simulink model "NL_Simulation"  (R2018b)
settings: Solver=VariableStepAuto  StartTime=0.0  StopTime=12.4  FixedStep=0.01
model workspace: external: MAT-File /home/abhineet/Research/Nonlinear_Model/Simulation_6dof/NL_Sim/setup_NL.mat (data not in the file)
values from neighbouring files (symbols this model uses):
  StateVals = SetInitial(Vinf,AeroType)    [setup_NL.m]
undefined symbols (not defined in the file or in its folder): AC, Mass
libraries: Tools_6dofSimulation x24, aerolibasang x3, dspmathops x3, shared6dofsys x2, shared6dof x2, aerolibatmos2 x1, sharedtransform x1, sharedutil x1
(part 2 of 2)

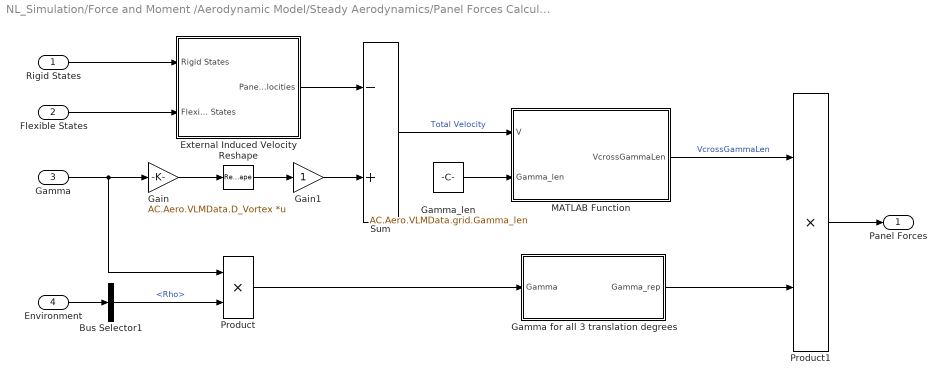
== system NL_Simulation/Force and Moment /Aerodynamic Model/Steady Aerodynamics/Panel Forces Calculation ==
  Rigid States : Inport
  Flexible States : Inport  Port=2
  Gamma : Inport  Port=3
  Environment : Inport  Port=4
  Bus Selector1 : BusSelector  OutputSignals=Rho
  External Induced Velocity : Subsystem
  Gain : Gain  Gain=AC.Aero.VLMData.D_Vortex  Multiplication=Matrix(K*u)
  Gain1 : Gain
  Gamma for all 3 translation degrees : MATLAB Function  TreatAsAtomicUnit=on
  Gamma_len : Constant  Value=AC.Aero.VLMData.grid.Gamma_len
  MATLAB Function : MATLAB Function  TreatAsAtomicUnit=on
  Product : Product
  Product1 : Product
  Reshape : Reshape  OutputDimensionality=Customize  OutputDimensions=[3,AC.Aero.NumPanels]
  Sum : Sum  Inputs=-+
  Panel Forces : Outport
  wires:
  Rigid States/1 -> External Induced Velocity/1(Rigid States)
  Flexible States/1 -> External Induced Velocity/2(Flexible States)
  External Induced Velocity/1(Panel Velocities) -> Sum/1
  Environment/1 -> Bus Selector1/1
  Gain/1 -> Reshape/1
  Reshape/1 -> Gain1/1
  Gamma/1 -> Gain/1, Product/1
  Sum/1 -> MATLAB Function/1(V)  "Total Velocity"
  Gamma_len/1 -> MATLAB Function/2(Gamma_len)
  Bus Selector1/1 -> Product/2  "<Rho>"
  Product/1 -> Gamma for all 3 translation degrees/1(Gamma)
  Gamma for all 3 translation degrees/1(Gamma_rep) -> Product1/2
  Product1/1 -> Panel Forces/1
  MATLAB Function/1(VcrossGammaLen) -> Product1/1  "VcrossGammaLen"
  Gain1/1 -> Sum/2

== system NL_Simulation/Force and Moment /Aerodynamic Model/Steady Aerodynamics/Total Wash ==
  note: The rigid body states are first transformed into Aerodynamic Axes and used to calculate total wash. Note that the calculated total wash is same as the internal wash generated by the vortices.
  Rigid States : Inport
  Flexible States : Inport  Port=2
  Bus Selector : BusSelector  OutputSignals=Vb,Omegab
  Flexible defections : Subsystem
  Gain : Gain  Gain=[-1,1,-1]
  Gain1 : Gain  Gain=[-1,1,-1]
  Repmat function : MATLAB Function  TreatAsAtomicUnit=on  mask{NumPanels=AC.Aero.NumPanels}
      mask prompts: NumPanels "Number of Panels"
      mask init:
      | % NumPanels = 888;
  Sum : Sum  Inputs=+++
  Vel_Omega : Subsystem
  Total  Wash : Outport
  wires:
  Rigid States/1 -> Bus Selector/1
  Bus Selector/1 -> Gain/1  "<Vb>"
  Bus Selector/2 -> Gain1/1  "<Omegab>"
  Vel_Omega/1(Omegacrossr) -> Sum/2
  Gain/1 -> Repmat function/1(V)
  Gain1/1 -> Vel_Omega/1(Omegab)
  Flexible States/1 -> Flexible defections/1(Flexible States)
  Flexible defections/1(Del_r_flex) -> Vel_Omega/2(Del_r_flex)
  Flexible defections/2(Del_v_flex) -> Sum/3
  Sum/1 -> Total  Wash/1
  Repmat function/1(Vrepmat) -> Sum/1

== system NL_Simulation/Force and Moment /Aerodynamic Model/Steady Aerodynamics/Vortex Strength ==
  Flexible States : Inport
  Normal wash : Inport  Port=2
  AIC Calculation : Subsystem
  Product : Product  Multiplication=Matrix(*)
  Gamma : Outport
  wires:
  Product/1 -> Gamma/1
  Flexible States/1 -> AIC Calculation/1(Flexible States)
  AIC Calculation/1(AIC) -> Product/1
  Normal wash/1 -> Product/2  "Normal wash"

== system NL_Simulation/Force and Moment /Aerodynamic Model/Unsteady Aerodynamics/Normal Forces ==
  Normal Wash Derivatives : Inport
  Rigid States : Inport  Port=2
  Gain : Gain  Gain=AC.Aero.DLMData.A1  Multiplication=Matrix(K*u)
  Gain1 : Gain  Gain=AC.Aero.DLMData.Clag  Multiplication=Matrix(K*u)
  MACby2V : Subsystem
  Product : Product
  Subsystem1 : Subsystem
  Sum : Sum
  Normal Forces : Outport
  wires:
  Normal Wash Derivatives/1 -> Product/1
  Sum/1 -> Normal Forces/1
  Rigid States/1 -> MACby2V/1(Rigid States)
  MACby2V/1(MACby2V) -> Product/2, Subsystem1/2(b_over_V)
  Product/1 -> Subsystem1/1(Normal Wash Derivative), Gain/1
  Gain/1 -> Sum/1
  Subsystem1/1(Lag States) -> Gain1/1
  Gain1/1 -> Sum/2

== system NL_Simulation/Force and Moment /Aerodynamic Model/Unsteady Aerodynamics/Normal Wash Derivative ==
  Total Wash Derivative : Inport
  Constant : Constant  Value=AC.Aero.Nhat0
  Product : Product
  Sum : Sum  Inputs=+  CollapseMode=Specified dimension
  Transpose : Math  Operator=transpose  SaturateOnIntegerOverflow=on
  Normal Wash Derivative : Outport
  wires:
  Sum/1 -> Transpose/1
  Constant/1 -> Product/1
  Total Wash Derivative/1 -> Product/2
  Product/1 -> Sum/1
  Transpose/1 -> Normal Wash Derivative/1

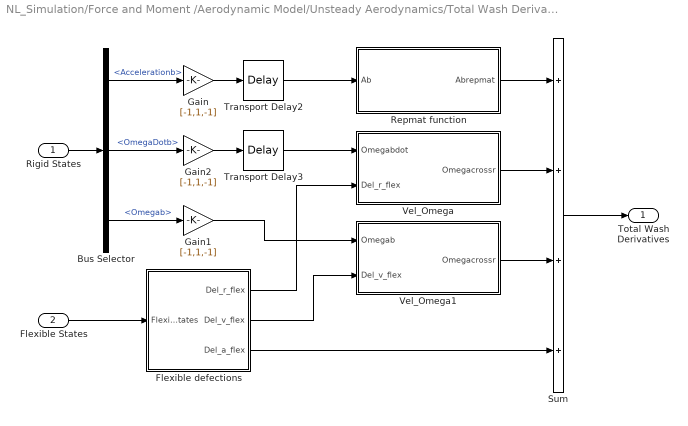
== system NL_Simulation/Force and Moment /Aerodynamic Model/Unsteady Aerodynamics/Total Wash Derivative ==
  Rigid States : Inport
  Flexible States : Inport  Port=2
  Bus Selector : BusSelector  OutputSignals=Accelerationb,OmegaDotb,Omegab
  Flexible defections : Subsystem
  Gain : Gain  Gain=[-1,1,-1]
  Gain1 : Gain  Gain=[-1,1,-1]
  Gain2 : Gain  Gain=[-1,1,-1]
  Repmat function : MATLAB Function  TreatAsAtomicUnit=on  mask{NumPanels=AC.Aero.NumPanels}
      mask prompts: NumPanels "Number of Panels"
      mask init:
      | % NumPanels = 888;
  Sum : Sum  Inputs=++++
  Transport Delay2 : TransportDelay  DelayTime=0.001  PadeOrder=2
  Transport Delay3 : TransportDelay  DelayTime=0.001  PadeOrder=2
  Vel_Omega : Subsystem
  Vel_Omega1 : Subsystem
  Total Wash Derivatives : Outport
  wires:
  Rigid States/1 -> Bus Selector/1
  Bus Selector/1 -> Gain/1  "<Accelerationb>"
  Vel_Omega/1(Omegacrossr) -> Sum/2
  Gain2/1 -> Transport Delay3/1
  Flexible States/1 -> Flexible defections/1(Flexible States)
  Sum/1 -> Total Wash Derivatives/1
  Repmat function/1(Abrepmat) -> Sum/1
  Bus Selector/2 -> Gain2/1  "<OmegaDotb>"
  Flexible defections/2(Del_v_flex) -> Vel_Omega1/2(Del_v_flex)
  Vel_Omega1/1(Omegacrossr) -> Sum/3
  Flexible defections/1(Del_r_flex) -> Vel_Omega/2(Del_r_flex)
  Gain/1 -> Transport Delay2/1
  Flexible defections/3(Del_a_flex) -> Sum/4
  Bus Selector/3 -> Gain1/1  "<Omegab>"
  Gain1/1 -> Vel_Omega1/1(Omegab)
  Transport Delay2/1 -> Repmat function/1(Ab)
  Transport Delay3/1 -> Vel_Omega/1(Omegabdot)

== system NL_Simulation/Sensors1/Sensors/Accelerometer Rigid/Vel_Omega ==
  Omegabdot : Inport
  Cross Product Matrix : Tools_6dofSimulation/Cross Product Matrix  SystemSampleTime=-1
  Demux : Demux  Outputs=3
  Product : Product  Multiplication=Matrix(*)
  rcg_sensor : Constant  Value=AC.SensorData.SensorAeroGrid
  Omegabcrossr : Outport
  wires:
  Omegabdot/1 -> Demux/1
  Product/1 -> Omegabcrossr/1
  Demux/2 -> Cross Product Matrix/2  "qdot"
  Demux/3 -> Cross Product Matrix/3  "rdot"
  Cross Product Matrix/1 -> Product/1
  rcg_sensor/1 -> Product/2
  Demux/1 -> Cross Product Matrix/1  "pdot"

== system NL_Simulation/Sensors1/Sensors/Accelerometer Rigid/Vel_Omega2 ==
  Omegabdot : Inport
  Cross Product Matrix : Tools_6dofSimulation/Cross Product Matrix  SystemSampleTime=-1
  Demux : Demux  Outputs=3
  Product : Product  Multiplication=Matrix(*)
  Product1 : Product  Multiplication=Matrix(*)
  rcg_sensor : Constant  Value=AC.SensorData.SensorAeroGrid
  Omegabcrossr : Outport
  wires:
  Omegabdot/1 -> Demux/1
  Demux/2 -> Cross Product Matrix/2  "qdot"
  Demux/3 -> Cross Product Matrix/3  "rdot"
  Cross Product Matrix/1 -> Product1/1, Product/1
  rcg_sensor/1 -> Product/2
  Demux/1 -> Cross Product Matrix/1  "pdot"
  Product/1 -> Product1/2
  Product1/1 -> Omegabcrossr/1

== system NL_Simulation/Sensors1/Sensors/Accelerometers/Flexible defections ==
  Flexible States : Inport
  Bus Selector1 : BusSelector  OutputSignals=EtaFlex,EtaFlexdot,EtaFlexdotdot
  Phif_Translation : Constant  Value=AC.ModalStruc.Phif_aero_sensor_Trans  VectorParams1D=off
  Product1 : Product  Multiplication=Matrix(*)
  Product2 : Product  Multiplication=Matrix(*)
  Product3 : Product  Multiplication=Matrix(*)
  Reshape1 : Reshape  OutputDimensionality=Customize  OutputDimensions=[3,AC.SensorData.NumSensors]
  Reshape2 : Reshape  OutputDimensionality=Customize  OutputDimensions=[3,AC.SensorData.NumSensors]
  Reshape3 : Reshape  OutputDimensionality=Customize  OutputDimensions=[3,AC.SensorData.NumSensors]
  Del_r_flex : Outport
  Del_v_flex : Outport  Port=2
  Del_a_flex : Outport  Port=3
  wires:
  Product1/1 -> Reshape1/1
  Bus Selector1/2 -> Product2/2  "<EtaFlexdot>"
  Reshape1/1 -> Del_r_flex/1
  Flexible States/1 -> Bus Selector1/1
  Product2/1 -> Reshape2/1
  Phif_Translation/1 -> Product3/1, Product2/1, Product1/1
  Bus Selector1/1 -> Product1/2  "<EtaFlex>"
  Reshape2/1 -> Del_v_flex/1
  Bus Selector1/3 -> Product3/2  "<EtaFlexdotdot>"
  Product3/1 -> Reshape3/1
  Reshape3/1 -> Del_a_flex/1

== system NL_Simulation/Sensors1/Sensors/Accelerometers/Subsystem ==
  In1 : Inport
  Bus Selector1 : BusSelector  OutputSignals=EtaFlex
  Gain : Gain  Gain=AC.ModalStruc.Phif_aero_sensor_Rot  Multiplication=Matrix(K*u)
  Normalization : dspmathops/Normalization  NormType=2-norm  Bias=1e-10  NormOver=Each column  Dimension=1  roundingMode=Floor  overflowMode=off  accumDataTypeStr=Inherit: Same as product output  accumLastDataTypeStr=Inherit: Same as product output  outputDataTypeStr=Inherit: Same as product output  outputMin=[]  outputMax=[]  outputLastDataTypeStr=Inherit: Same as product output
      settings: SourceProductName=DSP System Toolbox
  Reshape : Reshape  OutputDimensionality=Customize  OutputDimensions=[3,AC.SensorData.NumSensors]
  SensorOrient : Constant  Value=AC.SensorData.SensorOrientation
  Sum1 : Sum
  Out1 : Outport
  wires:
  SensorOrient/1 -> Sum1/2
  Normalization/1 -> Out1/1
  Reshape/1 -> Sum1/1
  In1/1 -> Bus Selector1/1
  Sum1/1 -> Normalization/1
  Gain/1 -> Reshape/1
  Bus Selector1/1 -> Gain/1  "<EtaFlex>"

== system NL_Simulation/Sensors1/Sensors/Accelerometers/Vel_Omega ==
  Omegabdot : Inport
  Del_r_flex : Inport  Port=2
  Cross Product Matrix : Tools_6dofSimulation/Cross Product Matrix  SystemSampleTime=-1
  Demux : Demux  Outputs=3
  Product : Product  Multiplication=Matrix(*)
  Sum : Sum
  rcg_sensor : Constant  Value=AC.SensorData.SensorAeroGrid
  Omegabcrossr : Outport
  wires:
  Omegabdot/1 -> Demux/1
  Product/1 -> Omegabcrossr/1
  Demux/2 -> Cross Product Matrix/2  "qdot"
  Demux/3 -> Cross Product Matrix/3  "rdot"
  Cross Product Matrix/1 -> Product/1
  Sum/1 -> Product/2
  Del_r_flex/1 -> Sum/1
  rcg_sensor/1 -> Sum/2
  Demux/1 -> Cross Product Matrix/1  "pdot"

== system NL_Simulation/Sensors1/Sensors/Accelerometers/Vel_Omega1 ==
  Omegab : Inport
  Del_v_flex : Inport  Port=2
  Cross Product Matrix : Tools_6dofSimulation/Cross Product Matrix  SystemSampleTime=-1
  Demux : Demux  Outputs=3
  Gain : Gain  Gain=2
  Product : Product  Multiplication=Matrix(*)
  TwoOmegabcrossrdot : Outport
  wires:
  Omegab/1 -> Demux/1
  Product/1 -> Gain/1
  Demux/2 -> Cross Product Matrix/2  "qdot"
  Demux/3 -> Cross Product Matrix/3  "rdot"
  Cross Product Matrix/1 -> Product/1
  Del_v_flex/1 -> Product/2
  Demux/1 -> Cross Product Matrix/1  "pdot"
  Gain/1 -> TwoOmegabcrossrdot/1

== system NL_Simulation/Sensors1/Sensors/Accelerometers/Vel_Omega2 ==
  Omegabdot : Inport
  Del_r_flex : Inport  Port=2
  Cross Product Matrix : Tools_6dofSimulation/Cross Product Matrix  SystemSampleTime=-1
  Demux : Demux  Outputs=3
  Product : Product  Multiplication=Matrix(*)
  Product1 : Product  Multiplication=Matrix(*)
  Sum : Sum
  rcg_sensor : Constant  Value=AC.SensorData.SensorAeroGrid
  Omegabcrossr : Outport
  wires:
  Omegabdot/1 -> Demux/1
  Demux/2 -> Cross Product Matrix/2  "qdot"
  Demux/3 -> Cross Product Matrix/3  "rdot"
  Cross Product Matrix/1 -> Product1/1, Product/1
  Sum/1 -> Product/2
  Del_r_flex/1 -> Sum/1
  rcg_sensor/1 -> Sum/2
  Demux/1 -> Cross Product Matrix/1  "pdot"
  Product/1 -> Product1/2
  Product1/1 -> Omegabcrossr/1

== system NL_Simulation/Flight Mechanics/Added Mass/Subsystem3/Normal Forces/MACby2V ==
  Rigid States : Inport
  Bus Selector : BusSelector  OutputSignals=Vb
  Constant : Constant  Value=AC.Aero.MAC
  Gain : Gain  Gain=.5
  Product : Product  Inputs=*/
  Vs Calculation : Subsystem
  MACby2V : Outport
  wires:
  Vs Calculation/1(Vs) -> Product/2
  Rigid States/1 -> Bus Selector/1
  Product/1 -> MACby2V/1
  Bus Selector/1 -> Vs Calculation/1(<Vb>)  "<Vb>"
  Constant/1 -> Gain/1
  Gain/1 -> Product/1

== system NL_Simulation/Flight Mechanics/Added Mass/Subsystem3/Normal Forces/Subsystem1 ==
  Normal Wash Derivative : Inport
  b_over_V : Inport  Port=2
  A_lag : Gain  Gain=AC.Aero.DLMData.Alag  Multiplication=Matrix(K*u)
  B_lag : Gain  Gain=AC.Aero.DLMData.Blag  Multiplication=Matrix(K*u)
  Lag : Integrator  InitialCondition=zeros(1776,1)
  Product : Product  Inputs=/*
  Sum : Sum  Inputs=|++
  Lag States : Outport
  wires:
  Normal Wash Derivative/1 -> B_lag/1
  B_lag/1 -> Sum/1
  Sum/1 -> Lag/1
  Lag/1 -> Product/2
  b_over_V/1 -> Product/1
  Product/1 -> A_lag/1, Lag States/1
  A_lag/1 -> Sum/2

== system NL_Simulation/Flight Mechanics/Added Mass/Subsystem3/Total Wash Derivative/Flexible defections ==
  Flexible States : Inport
  Bus Selector1 : BusSelector  OutputSignals=EtaFlex,EtaFlexdot,EtaFlexdotdot
  Phif_Translation : Constant  Value=AC.ModalStruc.Phif_aero_trans
  Product1 : Product  Multiplication=Matrix(*)
  Product2 : Product  Multiplication=Matrix(*)
  Product3 : Product  Multiplication=Matrix(*)
  Reshape1 : Reshape  OutputDimensionality=Customize  OutputDimensions=[3,AC.Aero.NumPanels]
  Reshape2 : Reshape  OutputDimensionality=Customize  OutputDimensions=[3,AC.Aero.NumPanels]
  Reshape3 : Reshape  OutputDimensionality=Customize  OutputDimensions=[3,AC.Aero.NumPanels]
  Transport Delay3 : TransportDelay  DelayTime=0.001  PadeOrder=2
  Del_r_flex : Outport
  Del_v_flex : Outport  Port=2
  Del_a_flex : Outport  Port=3
  wires:
  Product1/1 -> Reshape1/1
  Bus Selector1/2 -> Product2/2  "<EtaFlexdot>"
  Reshape1/1 -> Del_r_flex/1
  Flexible States/1 -> Bus Selector1/1
  Product2/1 -> Reshape2/1
  Bus Selector1/1 -> Product1/2  "<EtaFlex>"
  Reshape2/1 -> Del_v_flex/1
  Phif_Translation/1 -> Product3/1, Product2/1, Product1/1
  Bus Selector1/3 -> Transport Delay3/1  "<EtaFlexdotdot>"
  Product3/1 -> Reshape3/1
  Reshape3/1 -> Del_a_flex/1
  Transport Delay3/1 -> Product3/2

== system NL_Simulation/Flight Mechanics/Added Mass/Subsystem3/Total Wash Derivative/Vel_Omega ==
  Omegabdot : Inport
  Del_r_flex : Inport  Port=2
  Cross Product Matrix : Tools_6dofSimulation/Cross Product Matrix  SystemSampleTime=-1
  Demux : Demux  Outputs=3
  Product : Product  Multiplication=Matrix(*)
  Sum : Sum
  rcg_colloc : Constant  Value=AC.Aero.VLMData.grid.r_cgcolloc
  Omegacrossr : Outport
  wires:
  Omegabdot/1 -> Demux/1
  Product/1 -> Omegacrossr/1
  Demux/2 -> Cross Product Matrix/2  "q"
  Demux/3 -> Cross Product Matrix/3  "r"
  Cross Product Matrix/1 -> Product/1
  Sum/1 -> Product/2
  Del_r_flex/1 -> Sum/1
  rcg_colloc/1 -> Sum/2
  Demux/1 -> Cross Product Matrix/1  "p"

== system NL_Simulation/Flight Mechanics/Added Mass/Subsystem3/Total Wash Derivative/Vel_Omega1 ==
  Omegab : Inport
  Del_v_flex : Inport  Port=2
  Cross Product Matrix : Tools_6dofSimulation/Cross Product Matrix  SystemSampleTime=-1
  Demux : Demux  Outputs=3
  Product : Product  Multiplication=Matrix(*)
  Omegacrossr : Outport
  wires:
  Omegab/1 -> Demux/1
  Product/1 -> Omegacrossr/1
  Demux/2 -> Cross Product Matrix/2  "q"
  Demux/3 -> Cross Product Matrix/3  "r"
  Cross Product Matrix/1 -> Product/1
  Del_v_flex/1 -> Product/2
  Demux/1 -> Cross Product Matrix/1  "p"

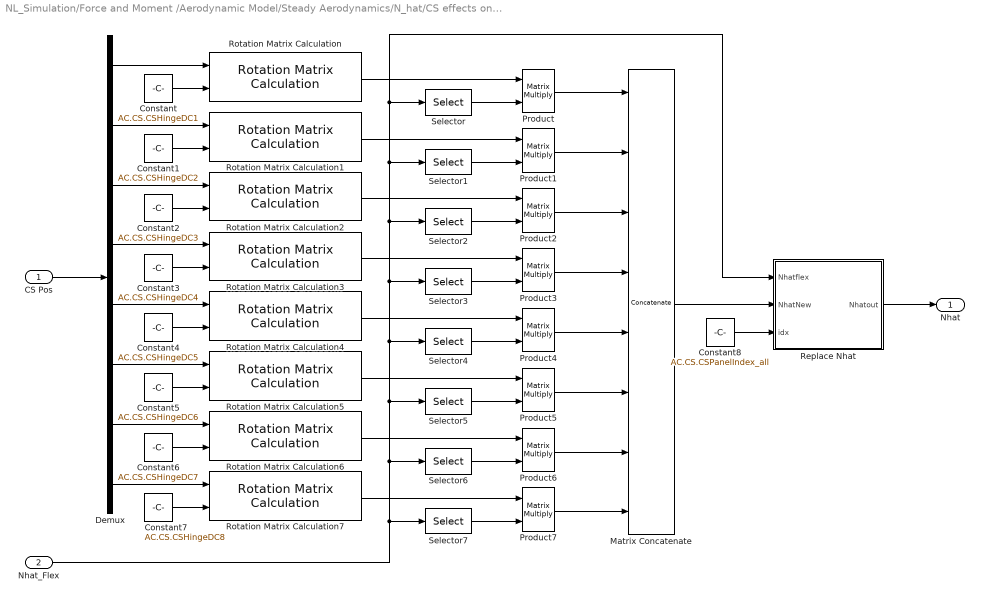
== system NL_Simulation/Force and Moment /Aerodynamic Model/Steady Aerodynamics/N_hat/CS effects on normal vectors ==
  CS Pos : Inport
  Nhat_Flex : Inport  Port=2
  Constant : Constant  Value=AC.CS.CSHingeDC1
  Constant1 : Constant  Value=AC.CS.CSHingeDC2
  Constant2 : Constant  Value=AC.CS.CSHingeDC3
  Constant3 : Constant  Value=AC.CS.CSHingeDC4
  Constant4 : Constant  Value=AC.CS.CSHingeDC5
  Constant5 : Constant  Value=AC.CS.CSHingeDC6
  Constant6 : Constant  Value=AC.CS.CSHingeDC7
  Constant7 : Constant  Value=AC.CS.CSHingeDC8
  Constant8 : Constant  Value=AC.CS.CSPanelIndex_all
  Demux : Demux  Outputs=8
  Matrix Concatenate : Concatenate  NumInputs=8  Mode=Multidimensional array  ConcatenateDimension=2
  Product{,1..7} (8 alike) : Product  Multiplication=Matrix(*)
  Replace Nhat : MATLAB Function  TreatAsAtomicUnit=on
  Rotation Matrix Calculation{,1..7} (8 alike) : Tools_6dofSimulation/Rotation Matrix Calculation  SystemSampleTime=-1
  Selector : Selector  NumberOfDimensions=2  InputPortWidth=3  IndexOptions=Select all,Index vector (dialog)  Indices=[1 3],AC.CS.CSPanelIndex1  OutputSizes=1,1
  Selector1 : Selector  NumberOfDimensions=2  InputPortWidth=3  IndexOptions=Select all,Index vector (dialog)  Indices=[1 3],AC.CS.CSPanelIndex2  OutputSizes=1,1
  Selector2 : Selector  NumberOfDimensions=2  InputPortWidth=3  IndexOptions=Select all,Index vector (dialog)  Indices=[1 3],AC.CS.CSPanelIndex3  OutputSizes=1,1
  Selector3 : Selector  NumberOfDimensions=2  InputPortWidth=3  IndexOptions=Select all,Index vector (dialog)  Indices=[1 3],AC.CS.CSPanelIndex4  OutputSizes=1,1
  Selector4 : Selector  NumberOfDimensions=2  InputPortWidth=3  IndexOptions=Select all,Index vector (dialog)  Indices=[1 3],AC.CS.CSPanelIndex5  OutputSizes=1,1
  Selector5 : Selector  NumberOfDimensions=2  InputPortWidth=3  IndexOptions=Select all,Index vector (dialog)  Indices=[1 3],AC.CS.CSPanelIndex6  OutputSizes=1,1
  Selector6 : Selector  NumberOfDimensions=2  InputPortWidth=3  IndexOptions=Select all,Index vector (dialog)  Indices=[1 3],AC.CS.CSPanelIndex7  OutputSizes=1,1
  Selector7 : Selector  NumberOfDimensions=2  InputPortWidth=3  IndexOptions=Select all,Index vector (dialog)  Indices=[1 3],AC.CS.CSPanelIndex8  OutputSizes=1,1
  Nhat : Outport
  wires:
  CS Pos/1 -> Demux/1
  Demux/1 -> Rotation Matrix Calculation/1
  Demux/2 -> Rotation Matrix Calculation1/1
  Demux/3 -> Rotation Matrix Calculation2/1
  Demux/4 -> Rotation Matrix Calculation3/1
  Demux/5 -> Rotation Matrix Calculation4/1
  Demux/6 -> Rotation Matrix Calculation5/1
  Demux/7 -> Rotation Matrix Calculation6/1
  Demux/8 -> Rotation Matrix Calculation7/1
  Constant/1 -> Rotation Matrix Calculation/2
  Constant1/1 -> Rotation Matrix Calculation1/2
  Constant2/1 -> Rotation Matrix Calculation2/2
  Constant3/1 -> Rotation Matrix Calculation3/2
  Constant4/1 -> Rotation Matrix Calculation4/2
  Constant5/1 -> Rotation Matrix Calculation5/2
  Constant6/1 -> Rotation Matrix Calculation6/2
  Constant7/1 -> Rotation Matrix Calculation7/2
  Rotation Matrix Calculation/1 -> Product/1
  Rotation Matrix Calculation1/1 -> Product1/1
  Rotation Matrix Calculation2/1 -> Product2/1
  Rotation Matrix Calculation3/1 -> Product3/1
  Rotation Matrix Calculation4/1 -> Product4/1
  Rotation Matrix Calculation6/1 -> Product6/1
  Rotation Matrix Calculation7/1 -> Product7/1
  Nhat_Flex/1 -> Replace Nhat/1(Nhatflex), Selector/1, Selector1/1, Selector2/1, Selector3/1, Selector4/1, Selector5/1, Selector6/1, Selector7/1
  Selector/1 -> Product/2
  Selector1/1 -> Product1/2
  Selector2/1 -> Product2/2
  Selector3/1 -> Product3/2
  Selector4/1 -> Product4/2
  Rotation Matrix Calculation5/1 -> Product5/1
  Selector5/1 -> Product5/2
  Selector6/1 -> Product6/2
  Selector7/1 -> Product7/2
  Constant8/1 -> Replace Nhat/3(idx)
  Product1/1 -> Matrix Concatenate/2
  Product2/1 -> Matrix Concatenate/3
  Product3/1 -> Matrix Concatenate/4
  Product4/1 -> Matrix Concatenate/5
  Product5/1 -> Matrix Concatenate/6
  Product6/1 -> Matrix Concatenate/7
  Product7/1 -> Matrix Concatenate/8
  Replace Nhat/1(Nhatout) -> Nhat/1
  Product/1 -> Matrix Concatenate/1
  Matrix Concatenate/1 -> Replace Nhat/2(NhatNew)

== system NL_Simulation/Force and Moment /Aerodynamic Model/Steady Aerodynamics/Panel Forces Calculation/External Induced Velocity ==
  Rigid States : Inport
  Flexible States : Inport  Port=2
  Bus Selector : BusSelector  OutputSignals=Vb,Omegab
  Flexible defections : Subsystem
  Gain : Gain  Gain=[-1,1,-1]
  Gain1 : Gain  Gain=[-1,1,-1]
  Repmat function : MATLAB Function  TreatAsAtomicUnit=on  mask{NumPanels=AC.Aero.NumPanels}
      mask prompts: NumPanels "Number of Panels"
      mask init:
      | % NumPanels = 888;
  Sum : Sum  Inputs=+++
  Vel_Omega : Subsystem
  Panel Velocities : Outport
  wires:
  Flexible defections/2(Del_v_flex) -> Sum/3
  Repmat function/1(Vrepmat) -> Sum/1
  Vel_Omega/1(Omegacrossr) -> Sum/2
  Flexible defections/1(Del_r_flex) -> Vel_Omega/2(Del_r_flex)
  Rigid States/1 -> Bus Selector/1
  Gain1/1 -> Vel_Omega/1(Omegab)
  Flexible States/1 -> Flexible defections/1(Flexible States)
  Bus Selector/2 -> Gain1/1  "<Omegab>"
  Bus Selector/1 -> Gain/1  "<Vb>"
  Gain/1 -> Repmat function/1(V)
  Sum/1 -> Panel Velocities/1

== system NL_Simulation/Force and Moment /Aerodynamic Model/Steady Aerodynamics/Total Wash/Flexible defections ==
  Flexible States : Inport
  Bus Selector1 : BusSelector  OutputSignals=EtaFlex,EtaFlexdot
  Phif_Translation : Constant  Value=AC.ModalStruc.Phif_aero_trans
  Product1 : Product  Multiplication=Matrix(*)
  Product2 : Product  Multiplication=Matrix(*)
  Reshape : Reshape  OutputDimensionality=Column vector (2-D)
  Reshape1 : Reshape  OutputDimensionality=Customize  OutputDimensions=[3,AC.Aero.NumPanels]
  Reshape2 : Reshape  OutputDimensionality=Customize  OutputDimensions=[3,AC.Aero.NumPanels]
  Reshape3 : Reshape  OutputDimensionality=Column vector (2-D)
  Del_r_flex : Outport
  Del_v_flex : Outport  Port=2
  wires:
  Product1/1 -> Reshape1/1
  Bus Selector1/2 -> Reshape3/1  "<EtaFlexdot>"
  Reshape1/1 -> Del_r_flex/1
  Flexible States/1 -> Bus Selector1/1
  Product2/1 -> Reshape2/1
  Phif_Translation/1 -> Product2/1, Product1/1
  Bus Selector1/1 -> Reshape/1  "<EtaFlex>"
  Reshape2/1 -> Del_v_flex/1
  Reshape/1 -> Product1/2
  Reshape3/1 -> Product2/2

== system NL_Simulation/Force and Moment /Aerodynamic Model/Steady Aerodynamics/Total Wash/Vel_Omega ==
  Omegab : Inport
  Del_r_flex : Inport  Port=2
  Cross Product Matrix : Tools_6dofSimulation/Cross Product Matrix  SystemSampleTime=-1
  Demux : Demux  Outputs=3
  Product : Product  Multiplication=Matrix(*)
  Sum : Sum
  rcg_colloc : Constant  Value=AC.Aero.VLMData.grid.r_cgcolloc
  Omegacrossr : Outport
  wires:
  Omegab/1 -> Demux/1
  Product/1 -> Omegacrossr/1
  Demux/2 -> Cross Product Matrix/2  "q"
  Demux/3 -> Cross Product Matrix/3  "r"
  Cross Product Matrix/1 -> Product/1
  Sum/1 -> Product/2
  Del_r_flex/1 -> Sum/1
  rcg_colloc/1 -> Sum/2
  Demux/1 -> Cross Product Matrix/1  "p"

== system NL_Simulation/Force and Moment /Aerodynamic Model/Steady Aerodynamics/Vortex Strength/AIC Calculation ==
  note: The effect of flexible deflection of the aircraft on the AIC matrix itself is calculated here.
  Flexible States : Inport
  AIC due to Flex : Subsystem  Commented=on
  "Ainv0 " : Constant  Value=AC.Aero.VLMData.Ainv0
  Bus Selector : BusSelector  OutputSignals=EtaFlex
  Sum : Sum
  AIC : Outport
  wires:
  Sum/1 -> AIC/1  "AIC"
  "Ainv0 "/1 -> Sum/1
  Flexible States/1 -> Bus Selector/1
  Bus Selector/1 -> AIC due to Flex/1(Eta_Flex)  "<EtaFlex>"
  AIC due to Flex/1(AIC_Flex) -> Sum/2

== system NL_Simulation/Force and Moment /Aerodynamic Model/Unsteady Aerodynamics/Normal Forces/MACby2V ==
  Rigid States : Inport
  Bus Selector : BusSelector  OutputSignals=Vb
  Constant : Constant  Value=AC.Aero.MAC
  Gain : Gain  Gain=.5
  Product : Product  Inputs=*/
  Vs Calculation : Subsystem
  MACby2V : Outport
  wires:
  Vs Calculation/1(Vs) -> Product/2
  Rigid States/1 -> Bus Selector/1
  Product/1 -> MACby2V/1
  Bus Selector/1 -> Vs Calculation/1(<Vb>)  "<Vb>"
  Constant/1 -> Gain/1
  Gain/1 -> Product/1

== system NL_Simulation/Force and Moment /Aerodynamic Model/Unsteady Aerodynamics/Normal Forces/Subsystem1 ==
  Normal Wash Derivative : Inport
  b_over_V : Inport  Port=2
  A_lag : Gain  Gain=AC.Aero.DLMData.Alag  Multiplication=Matrix(K*u)
  B_lag : Gain  Gain=AC.Aero.DLMData.Blag  Multiplication=Matrix(K*u)
  Lag : Integrator  InitialCondition=zeros(1776,1)
  Product : Product  Inputs=/*
  Sum : Sum  Inputs=|++
  Lag States : Outport
  wires:
  Normal Wash Derivative/1 -> B_lag/1
  B_lag/1 -> Sum/1
  Sum/1 -> Lag/1
  Lag/1 -> Product/2
  b_over_V/1 -> Product/1
  Product/1 -> A_lag/1, Lag States/1
  A_lag/1 -> Sum/2

== system NL_Simulation/Force and Moment /Aerodynamic Model/Unsteady Aerodynamics/Total Wash Derivative/Flexible defections ==
  Flexible States : Inport
  Bus Selector1 : BusSelector  OutputSignals=EtaFlex,EtaFlexdot,EtaFlexdotdot
  Phif_Translation : Constant  Value=AC.ModalStruc.Phif_aero_trans
  Product1 : Product  Multiplication=Matrix(*)
  Product2 : Product  Multiplication=Matrix(*)
  Product3 : Product  Multiplication=Matrix(*)
  Reshape1 : Reshape  OutputDimensionality=Customize  OutputDimensions=[3,AC.Aero.NumPanels]
  Reshape2 : Reshape  OutputDimensionality=Customize  OutputDimensions=[3,AC.Aero.NumPanels]
  Reshape3 : Reshape  OutputDimensionality=Customize  OutputDimensions=[3,AC.Aero.NumPanels]
  Transport Delay3 : TransportDelay  DelayTime=0.001  PadeOrder=2
  Del_r_flex : Outport
  Del_v_flex : Outport  Port=2
  Del_a_flex : Outport  Port=3
  wires:
  Product1/1 -> Reshape1/1
  Bus Selector1/2 -> Product2/2  "<EtaFlexdot>"
  Reshape1/1 -> Del_r_flex/1
  Flexible States/1 -> Bus Selector1/1
  Product2/1 -> Reshape2/1
  Bus Selector1/1 -> Product1/2  "<EtaFlex>"
  Reshape2/1 -> Del_v_flex/1
  Phif_Translation/1 -> Product3/1, Product2/1, Product1/1
  Bus Selector1/3 -> Transport Delay3/1  "<EtaFlexdotdot>"
  Product3/1 -> Reshape3/1
  Reshape3/1 -> Del_a_flex/1
  Transport Delay3/1 -> Product3/2

== system NL_Simulation/Force and Moment /Aerodynamic Model/Unsteady Aerodynamics/Total Wash Derivative/Vel_Omega ==
  Omegabdot : Inport
  Del_r_flex : Inport  Port=2
  Cross Product Matrix : Tools_6dofSimulation/Cross Product Matrix  SystemSampleTime=-1
  Demux : Demux  Outputs=3
  Product : Product  Multiplication=Matrix(*)
  Sum : Sum
  rcg_colloc : Constant  Value=AC.Aero.VLMData.grid.r_cgcolloc
  Omegacrossr : Outport
  wires:
  Omegabdot/1 -> Demux/1
  Product/1 -> Omegacrossr/1
  Demux/2 -> Cross Product Matrix/2  "q"
  Demux/3 -> Cross Product Matrix/3  "r"
  Cross Product Matrix/1 -> Product/1
  Sum/1 -> Product/2
  Del_r_flex/1 -> Sum/1
  rcg_colloc/1 -> Sum/2
  Demux/1 -> Cross Product Matrix/1  "p"

== system NL_Simulation/Force and Moment /Aerodynamic Model/Unsteady Aerodynamics/Total Wash Derivative/Vel_Omega1 ==
  Omegab : Inport
  Del_v_flex : Inport  Port=2
  Cross Product Matrix : Tools_6dofSimulation/Cross Product Matrix  SystemSampleTime=-1
  Demux : Demux  Outputs=3
  Product : Product  Multiplication=Matrix(*)
  Omegacrossr : Outport
  wires:
  Omegab/1 -> Demux/1
  Product/1 -> Omegacrossr/1
  Demux/2 -> Cross Product Matrix/2  "q"
  Demux/3 -> Cross Product Matrix/3  "r"
  Cross Product Matrix/1 -> Product/1
  Del_v_flex/1 -> Product/2
  Demux/1 -> Cross Product Matrix/1  "p"

== system NL_Simulation/Flight Mechanics/Added Mass/Subsystem3/Normal Forces/MACby2V/Vs Calculation ==
  <Vb> : Inport
  Demux : Demux  Outputs=3
  Product : Product
  Product1 : Product
  Product2 : Product
  Sqrt : Sqrt  SaturateOnIntegerOverflow=on
  Sum : Sum  Inputs=+++
  Vs : Outport
  wires:
  Sum/1 -> Sqrt/1
  Product/1 -> Sum/1
  Demux/3 -> Product2/1, Product2/2
  <Vb>/1 -> Demux/1
  Product1/1 -> Sum/2
  Demux/2 -> Product1/1, Product1/2
  Product2/1 -> Sum/3
  Sqrt/1 -> Vs/1
  Demux/1 -> Product/1, Product/2

== system NL_Simulation/Force and Moment /Aerodynamic Model/Steady Aerodynamics/Panel Forces Calculation/External Induced Velocity/Flexible defections ==
  Flexible States : Inport
  Bus Selector1 : BusSelector  OutputSignals=EtaFlex,EtaFlexdot
  Phif_Translation : Constant  Value=AC.ModalStruc.Phif_aero_trans
  Product1 : Product  Multiplication=Matrix(*)
  Product2 : Product  Multiplication=Matrix(*)
  Reshape1 : Reshape  OutputDimensionality=Customize  OutputDimensions=[3,AC.Aero.NumPanels]
  Reshape2 : Reshape  OutputDimensionality=Customize  OutputDimensions=[3,AC.Aero.NumPanels]
  Del_r_flex : Outport
  Del_v_flex : Outport  Port=2
  wires:
  Product1/1 -> Reshape1/1
  Bus Selector1/2 -> Product2/2  "<EtaFlexdot>"
  Reshape1/1 -> Del_r_flex/1
  Flexible States/1 -> Bus Selector1/1
  Product2/1 -> Reshape2/1
  Phif_Translation/1 -> Product2/1, Product1/1
  Bus Selector1/1 -> Product1/2  "<EtaFlex>"
  Reshape2/1 -> Del_v_flex/1

== system NL_Simulation/Force and Moment /Aerodynamic Model/Steady Aerodynamics/Panel Forces Calculation/External Induced Velocity/Vel_Omega ==
  Omegab : Inport
  Del_r_flex : Inport  Port=2
  Cross Product Matrix : Tools_6dofSimulation/Cross Product Matrix  SystemSampleTime=-1
  Demux : Demux  Outputs=3
  Product : Product  Multiplication=Matrix(*)
  Sum : Sum
  rcg_vortex : Constant  Value=AC.Aero.VLMData.grid.r_cgvortex
  Omegacrossr : Outport
  wires:
  Omegab/1 -> Demux/1
  Product/1 -> Omegacrossr/1
  Demux/2 -> Cross Product Matrix/2  "q"
  Demux/3 -> Cross Product Matrix/3  "r"
  Cross Product Matrix/1 -> Product/1
  Sum/1 -> Product/2
  Del_r_flex/1 -> Sum/1
  rcg_vortex/1 -> Sum/2
  Demux/1 -> Cross Product Matrix/1  "p"

== system NL_Simulation/Force and Moment /Aerodynamic Model/Steady Aerodynamics/Vortex Strength/AIC Calculation/AIC due to Flex ==
  Eta_Flex : Inport
  Demux : Demux  Outputs=5
  Gain : Gain  Gain=AC.Aero.VLMData.Ainv_eta.Ainv_eta_R{1}
  Gain1 : Gain  Gain=AC.Aero.VLMData.Ainv_eta.Ainv_eta_L{1}  Multiplication=Matrix(K*u)
  Gain2 : Gain  Gain=AC.Aero.VLMData.Ainv_eta.Ainv_eta_R{2}
  Gain3 : Gain  Gain=AC.Aero.VLMData.Ainv_eta.Ainv_eta_L{2}  Multiplication=Matrix(K*u)
  Gain4 : Gain  Gain=AC.Aero.VLMData.Ainv_eta.Ainv_eta_R{3}
  Gain5 : Gain  Gain=AC.Aero.VLMData.Ainv_eta.Ainv_eta_L{3}  Multiplication=Matrix(K*u)
  Gain6 : Gain  Gain=AC.Aero.VLMData.Ainv_eta.Ainv_eta_R{4}
  Gain7 : Gain  Gain=AC.Aero.VLMData.Ainv_eta.Ainv_eta_L{4}  Multiplication=Matrix(K*u)
  Gain8 : Gain  Gain=AC.Aero.VLMData.Ainv_eta.Ainv_eta_R{5}
  Gain9 : Gain  Gain=AC.Aero.VLMData.Ainv_eta.Ainv_eta_L{5}  Multiplication=Matrix(K*u)
  Sum : Sum  Inputs=+++++
  AIC_Flex : Outport
  wires:
  Gain2/1 -> Gain3/1
  Gain8/1 -> Gain9/1
  ? -> ?
  Gain3/1 -> Sum/2
  Gain1/1 -> Sum/1
  Gain/1 -> Gain1/1
  Gain5/1 -> Sum/3
  Demux/3 -> Gain4/1  "eta3"
  Gain7/1 -> Sum/4
  Gain9/1 -> Sum/5
  Demux/5 -> Gain8/1  "eta2"
  Gain4/1 -> Gain5/1
  Demux/1 -> Gain/1  "eta1"
  Demux/2 -> Gain2/1  "eta2"
  Demux/4 -> Gain6/1  "eta1"
  Gain6/1 -> Gain7/1
  Sum/1 -> AIC_Flex/1
  Eta_Flex/1 -> Demux/1

== system NL_Simulation/Force and Moment /Aerodynamic Model/Unsteady Aerodynamics/Normal Forces/MACby2V/Vs Calculation ==
  <Vb> : Inport
  Demux : Demux  Outputs=3
  Product : Product
  Product1 : Product
  Product2 : Product
  Sqrt : Sqrt  SaturateOnIntegerOverflow=on
  Sum : Sum  Inputs=+++
  Vs : Outport
  wires:
  Sum/1 -> Sqrt/1
  Product/1 -> Sum/1
  Demux/3 -> Product2/1, Product2/2
  <Vb>/1 -> Demux/1
  Product1/1 -> Sum/2
  Demux/2 -> Product1/1, Product1/2
  Product2/1 -> Sum/3
  Sqrt/1 -> Vs/1
  Demux/1 -> Product/1, Product/2

== matlab function NL_Simulation/Force and Moment /Aerodynamic Model/Unsteady Aerodynamics/Total Wash Derivative/Repmat function ==
  data: Ab input; Abrepmat output; NumPanels parameter
function Abrepmat = fcn(Ab,NumPanels)
Abrepmat = repmat(Ab,1,NumPanels);
end

== matlab function NL_Simulation/Force and Moment /Aerodynamic Model/Steady Aerodynamics/Total Wash/Repmat function ==
  data: V input; Vrepmat output; NumPanels parameter
function Vrepmat = fcn(V,NumPanels)
Vrepmat = repmat(V,1,NumPanels);
end

== matlab function NL_Simulation/Force and Moment /Aerodynamic Model/Unsteady Aerodynamics/MATLAB Function ==
  data: nhat0 input; TotalForces output; NormalForces input
function TotalForces = fcn(nhat0,NormalForces)
%nhat0 = 3*888
%normalForce = 888*1
%TotalForce = 3*888;
Fx = zeros(888,1);
Fy = [zeros(552,1); NormalForces(553:888,1)];
Fz = [NormalForces(1:552,1); zeros(336,1)];

TotalForces = [Fx,Fy,Fz]'.*nhat0;

== matlab function NL_Simulation/Sensors1/Sensors/Accelerometers/Repmat function ==
  data: V input; Vrepmat output; NumSensors parameter
function Vrepmat = fcn(V,NumSensors)
Vrepmat = repmat(V,1,NumSensors);
end

== matlab function NL_Simulation/Sensors1/Sensors/IMUs/Repmat function ==
  data: V input; Vrepmat output; NumSensors parameter
function Vrepmat = fcn(V,NumSensors)
Vrepmat = repmat(V,1,NumSensors);
end

== matlab function NL_Simulation/Sensors1/Sensors/Accelerometer Rigid/Repmat function ==
  data: V input; Vrepmat output; NumSensors parameter
function Vrepmat = fcn(V,NumSensors)
Vrepmat = repmat(V,1,NumSensors);
end

== matlab function NL_Simulation/Flight Mechanics/Added Mass/Subsystem3/MATLAB Function ==
  data: nhat0 input; TotalForces output; NormalForces input
function TotalForces = fcn(nhat0,NormalForces)
%nhat0 = 3*888
%normalForce = 888*1
%TotalForce = 3*888;
Fx = zeros(888,1);
Fy = [zeros(552,1); NormalForces(553:888,1)];
Fz = [NormalForces(1:552,1); zeros(336,1)];

TotalForces = [Fx,Fy,Fz]'.*nhat0;

== matlab function NL_Simulation/Flight Mechanics/Added Mass/Subsystem3/Total Wash Derivative/Repmat function ==
  data: Ab input; Abrepmat output; NumPanels parameter
function Abrepmat = fcn(Ab,NumPanels)
Abrepmat = repmat(Ab,1,NumPanels);
end

== matlab function NL_Simulation/Sensors1/Accelerometer Rigid/Repmat function ==
  data: V input; Vrepmat output; NumSensors parameter
function Vrepmat = fcn(V,NumSensors)
Vrepmat = repmat(V,1,NumSensors);
end

== matlab function NL_Simulation/Force and Moment /Aerodynamic Model/Steady Aerodynamics/N_hat/CS effects on normal vectors/Replace Nhat ==
  data: Nhatflex input; Nhatout output; NhatNew input; idx input
function Nhatout = fcn(Nhatflex,NhatNew,idx)
Nhatout = Nhatflex;
Nhatout(:,idx) = NhatNew;

== matlab function NL_Simulation/Sensors1/Accelerometers/Repmat function ==
  data: AbTotal input; AbTotalrepmat output; NumSensors parameter
function AbTotalrepmat = fcn(AbTotal,NumSensors)
AbTotalrepmat = repmat(AbTotal,1,NumSensors);
end

== matlab function NL_Simulation/Force and Moment /Aerodynamic Model/Steady Aerodynamics/Panel Forces Calculation/External Induced Velocity/Repmat function ==
  data: V input; Vrepmat output; NumPanels parameter
function Vrepmat = fcn(V,NumPanels)
Vrepmat = repmat(V,1,NumPanels);
end

== matlab function NL_Simulation/Sensors1/IMUs/Repmat function ==
  data: V input; Vrepmat output; NumSensors parameter
function Vrepmat = fcn(V,NumSensors)
Vrepmat = repmat(V,1,NumSensors);
end

== matlab function NL_Simulation/Force and Moment /Aerodynamic Model/Steady Aerodynamics/Panel Forces Calculation/MATLAB Function ==
  data: V input; VcrossGammaLen output; Gamma_len input
function VcrossGammaLen = fcn(V,Gamma_len)
VcrossGammaLen = cross(V,Gamma_len,1);
end

== matlab function NL_Simulation/Force and Moment /Aerodynamic Model/Steady Aerodynamics/Panel Forces Calculation/Gamma for all 3 translation degrees ==
  data: Gamma input; Gamma_rep output
function Gamma_rep = fcn(Gamma)
Gamma_rep = repmat(Gamma,1,3)';
end

== matlab function NL_Simulation/Force and Moment /Total Forces and Moments/MATLAB Function ==
  data: R input; SumRcrossF output; F input
function SumRcrossF = fcn(R,F)
SumRcrossF = sum(cross(R,F),2);
end
